simulink model "simpleModel"  (R2018a)
settings: Solver=VariableStepAuto  StartTime=0.0  StopTime=100  RelTol=1e-3
settings Model: Creator=transmogrifier  LastModifiedBy=thedoctor

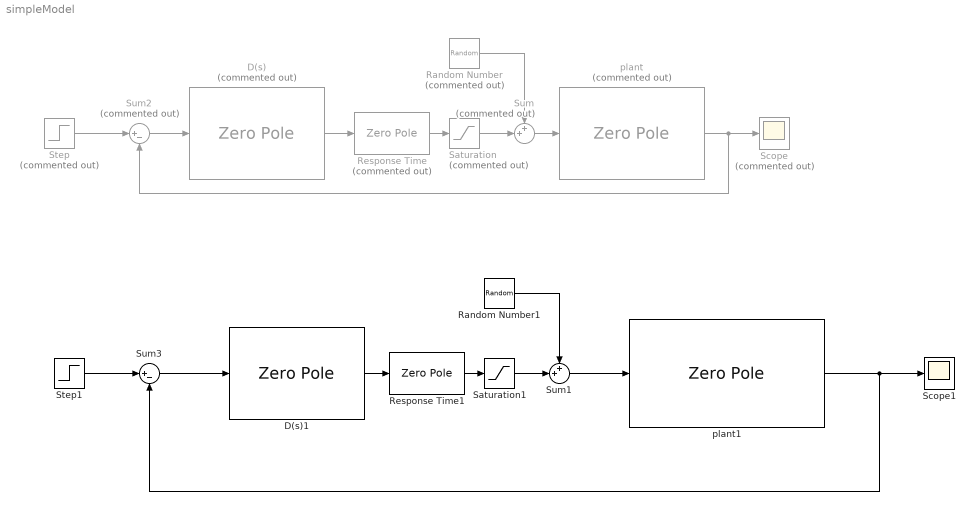
== system simpleModel ==
  D(s) : ZeroPole  Commented=on  Zeros=[-0.2668]  Poles=[-8]  Gain=[64.4]
  D(s)1 : ZeroPole  Zeros=[-0.2668]  Poles=[-26]  Gain=[1619]
  Random Number : RandomNumber  Commented=on  Variance=pi/48  SampleTime=0.1
  Random Number1 : RandomNumber  Variance=pi/48  SampleTime=0.1
  Response Time : ZeroPole  Commented=on  Zeros=[]  Poles=[-5]
  Response Time1 : ZeroPole  Zeros=[]  Poles=[-5]
  Saturation : Saturate  Commented=on  UpperLimit=pi/12  LowerLimit=-pi/12
  Saturation1 : Saturate  UpperLimit=pi/12  LowerLimit=-pi/12
  Scope : Scope  Commented=on
  Scope1 : Scope
  Step : Step  Commented=on  Time=0  After=4  SampleTime=0
  Step1 : Step  Time=0  After=4  SampleTime=0
  Sum : Sum  Commented=on  Inputs=++|
  Sum1 : Sum  Inputs=++|
  Sum2 : Sum  Commented=on  Inputs=|+-
  Sum3 : Sum  Inputs=|+-
  plant : ZeroPole  Commented=on  Zeros=[]  Poles=[0 0 -5/4]  Gain=[1.5]
  plant1 : ZeroPole  Zeros=[]  Poles=[0 0 -5/4]  Gain=[1.5/100]
  wires:
  Sum2/1 -> D(s)/1
  Step/1 -> Sum2/1
  plant/1 -> Sum2/2, Scope/1
  D(s)/1 -> Response Time/1
  Response Time/1 -> Saturation/1
  Random Number/1 -> Sum/1
  Saturation/1 -> Sum/2
  Sum/1 -> plant/1
  Sum3/1 -> D(s)1/1
  plant1/1 -> Sum3/2, Scope1/1
  Step1/1 -> Sum3/1
  Random Number1/1 -> Sum1/1
  Response Time1/1 -> Saturation1/1
  Saturation1/1 -> Sum1/2
  D(s)1/1 -> Response Time1/1
  Sum1/1 -> plant1/1
